simulink model "IO102simpleloopback"  (R2013a)
settings: Solver=FixedStepDiscrete  StartTime=0.0  StopTime=inf  RelTol=1e-3
libraries: speedgoatlib_IO102 x5, xpclib x2
settings Model: BufferReuse=off  Creator=dkuratli  LastModifiedBy=lab3
settings SolverCC: EnableConcurrentExecution=on
settings OptimizationCC: BlockReduction=off  OptimizeBlockIOStorage=off  BufferReuse=off  ExpressionFolding=off  LocalBlockOutputs=off
settings DebuggingCC: UnderspecifiedInitializationDetection=Simplified  StateNameClashWarn=none
settings HardwareCC: ProdIntDivRoundTo=Zero  ProdEndianess=LittleEndian  ProdHWDeviceType=Generic->32-bit x86 compatible
settings RTWCC: SystemTargetFile=xpctarget.tlc  TemplateMakefile=xpc_default_tmf  Description=Simulink Real-Time  RTWVerbose=off  ProcessScript=xpctarget_make_rtw_hook  RTWCompilerOptimization=On
settings xpcTargetCC: TargetFcnLib=ansi_tfl_table_tmw.mat  CodeReplacementLibrary=XPC_BLAS  ParMdlRefBuildCompliant=on  ConcurrentExecutionCompliant=on  CombineSignalStateStructs=off  MATLABClassNameForMDSCustomization=xpcAperiodicCustomization  GRTInterface=on  GenerateAllocFcn=off  xPCTaskExecutionProfile=off  xPCRL32EventNumber=5000  xPCLoadParamSetFile=off  xPCConcurrentTasks=off  xPCEnableSFAnimation=off

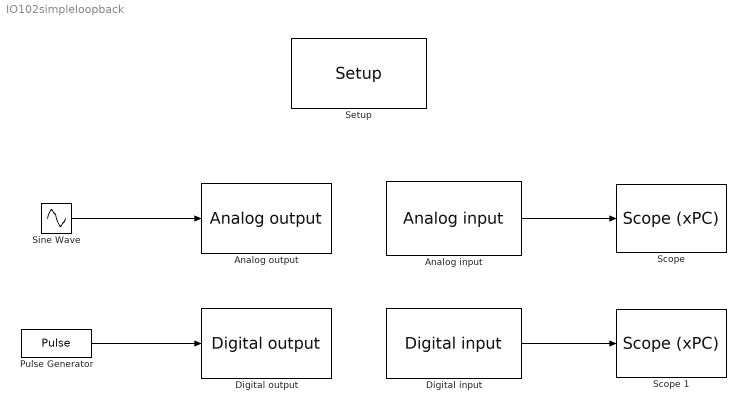
== system IO102simpleloopback ==
  Analog input : speedgoatlib_IO102/Analog input  id=1  channels=1  range=1  high_voltage=off  adCoupling=2  ts=100e-6  pciSlot=-1
  Analog output : speedgoatlib_IO102/Analog output  id=1  channels=1  range=1  ts=-1  pciSlot=-1
  Digital input : speedgoatlib_IO102/Digital input  id=1  channels=1  ts=100e-6  pciSlot=-1
  Digital output : speedgoatlib_IO102/Digital output  id=1  channels=1  ts=-1  pciSlot=-1
  Pulse Generator : DiscretePulseGenerator  Period=100  PulseWidth=50  SampleTime=100e-6
  "Scope " : xpclib/Misc./Scope (xPC)   scopeno=1  scopetype=Target  autostart=on  viewmode=Graphical redraw  formatstr='%15.6f'  grid=on  ylimits=[0,0]  nosamples=250  noprepostsamples=0  interleave=1  triggermode=FreeRun  triggersignal=1  trigsignalfromport=off  triggerlevel=0.0  triggerslope=Either  triggerscope=1  triggersample=0  filename=data.dat  mode=Lazy  writesize=512  autorestart=off  dynamicfilemode=off  maxwritefilesize=512*1024^2
  Scope 1 : xpclib/Misc./Scope (xPC)   scopeno=2  scopetype=Target  autostart=on  viewmode=Graphical redraw  formatstr='%15.6f'  grid=on  ylimits=[0,0]  nosamples=250  noprepostsamples=0  interleave=1  triggermode=FreeRun  triggersignal=1  trigsignalfromport=off  triggerlevel=0.0  triggerslope=Either  triggerscope=1  triggersample=0  filename=data.dat  mode=Lazy  writesize=512  autorestart=off  dynamicfilemode=off  maxwritefilesize=512*1024^2
  Setup : speedgoatlib_IO102/Setup  group=Module setup  id=1  range=+-10V  cal=on  pciSlot=-1  adChannelMode=Single-channel (enter channel number below)  adChannel=1  adCoupling=Single-ended  daChannel=[1]  daReset=[1]  daInitValue=[0]  diChannel=[1]  doChannel=[1]  doReset=[1]  doInitValue=[0]
  Sine Wave : Sin  Amplitude=10  Frequency=2*pi*500  SampleTime=100e-6
  wires:
  Sine Wave/1 -> Analog output/1
  Analog input/1 -> "Scope "/1
  Pulse Generator/1 -> Digital output/1
  Digital input/1 -> Scope 1/1
